simulink model "model_my_paper"  (R2024a)
settings: Solver=FixedStepAuto  StartTime=0.0  StopTime=40  FixedStep=0.01  RelTol=1e-3
undefined symbols (not defined in the file or in its folder): e0_0, e1_0, e2_0, e3_0, q0, vec
libraries: sharedtransform x8, dspsigops x3, aerolibsim3d x2, sharedutil x2, sim3dlib x1, aerolibutil x1
settings Model: Creator=bemran  LastModifiedBy=bemran

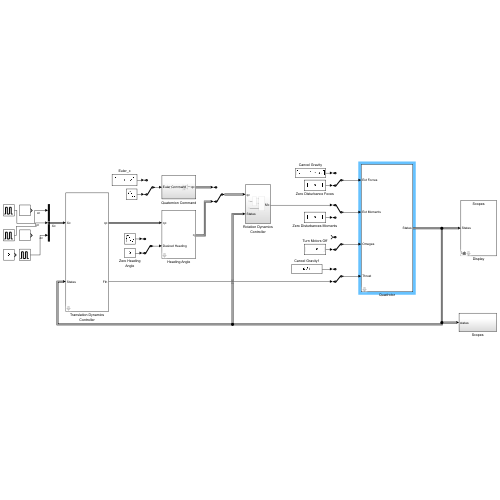
[thumbnail: Simulink's stored preview of the top-level diagram]
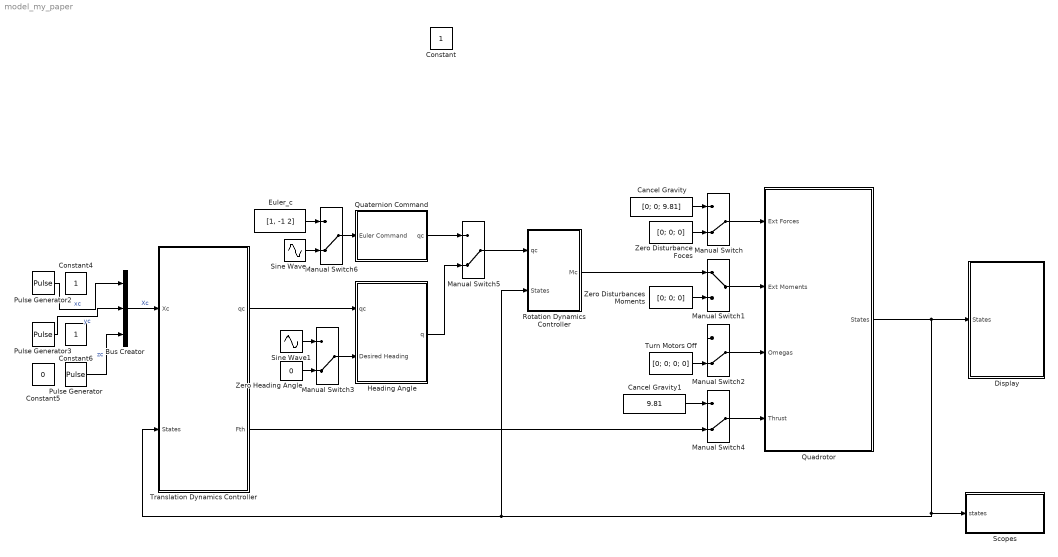
== system model_my_paper ==
  Bus Creator : BusCreator  Inputs=3
  Cancel Gravity : Constant  Value=[0; 0; 9.81]
  Cancel Gravity1 : Constant  Value=9.81
  Constant4 : Constant
  Constant5 : Constant  Value=0
  Constant6 : Constant
  Display : Subsystem  Variant=on  VariantControlMode=label  LabelModeActiveChoice=scopes  mask{VChoice=scopes}
      mask prompts: VChoice "Select method of display"
      mask init:
      | vssBlk = gcb;
      | choice = get_param(vssBlk,'VChoice');
      | if strcmp(choice,'animation')
      |     set_param(vssBlk, 'LabelModeActiveChoice', 'animation');
      | else
      |     set_param(vssBlk, 'LabelModeActiveChoice', 'scopes');
      | end
  Euler_c : Constant  Value=[1, -1 2]
  Heading Angle : Subsystem  mask{FallingSlewLimit=-1, HeadingRisingSlewLimit=1}
      mask prompts: FallingSlewLimit "Heading Falling Slew Limit"; HeadingRisingSlewLimit "Heading Rising Slew Limit"
      mask TypeOptions FallingSlewLimit: Rate Limiter/FallingSlewLimit
      mask TypeOptions HeadingRisingSlewLimit: Rate Limiter/RisingSlewLimit
  Manual Switch{,2..6} (6 alike) : ManualSwitch  CurrentSetting=0
  Manual Switch1 : ManualSwitch
  Pulse Generator : DiscretePulseGenerator  PulseType=Time based  Amplitude=-4  Period=20  PulseWidth=50
  Pulse Generator2 : DiscretePulseGenerator  PulseType=Time based  Amplitude=5  Period=30  PulseWidth=50  PhaseDelay=10
  Pulse Generator3 : DiscretePulseGenerator  PulseType=Time based  Amplitude=-3  Period=30  PulseWidth=50  PhaseDelay=-10
  Quadrotor : Subsystem  mask{mass=1, InertiaMatrix=eye(3), thrust_coff=1, drag_coff=0.1, arm_length=0.3, VelocityBodyInitialValues=zeros(3,1), PositionReferenceInitialValues=zeros(3,1), OmegaInitialValues=zeros(3,1), EulerInitialValues=zeros(3,1)}
      mask prompts: InertiaMatrix "Inertia Matrix"; thrust_coff "Thrust Coefficient"; drag_coff "Drag Coefficient"; arm_length "Arm Length"; VelocityBodyInitialValues "Velocity Body Initial Values"; PositionReferenceInitialValues "Position Reference Initial Values"; OmegaInitialValues "Omega Initial Values"; EulerInitialValues "Euler Initial Values"
      mask TypeOptions mass: 6DOF NWU Mixed/mass
      mask TypeOptions InertiaMatrix: 6DOF NWU Mixed/InertiaMatrix
      mask TypeOptions thrust_coff: Mixer/thrust_coff
      mask TypeOptions drag_coff: Mixer/drag_coff
      mask TypeOptions arm_length: Mixer/arm_length
      mask TypeOptions VelocityBodyInitialValues: 6DOF NWU Mixed/VelocityBodyInitialValues
      mask TypeOptions PositionReferenceInitialValues: 6DOF NWU Mixed/PositionReferenceInitialValues
      mask TypeOptions OmegaInitialValues: 6DOF NWU Mixed/OmegaInitialValues
      mask TypeOptions EulerInitialValues: 6DOF NWU Mixed/EulerInitialValues
  Quaternion Command : Subsystem
  Rotation Dynamics Controller : Subsystem
  Scopes : Subsystem  VariantControl=scopes
  Sine Wave : Sin  Amplitude=[1*pi;1*pi; 1*pi]  Frequency=[0.1, 0.05, 0.02]  Phase=[pi/6, pi/2, -pi/6]  SampleTime=0
  Sine Wave1 : Sin  Amplitude=2*pi  Frequency=0.1  SampleTime=0
  Translation Dynamics Controller : Subsystem
      mask DialogControl ParameterGroupVar Prompt: Desired Signal
      mask DialogControl Container3 Prompt: Control Signal
  Turn Motors Off : Constant  Value=[0; 0; 0; 0]
  Zero Disturbance Foces : Constant  Value=[0; 0; 0]
  Zero Disturbances Moments : Constant  Value=[0; 0; 0]
  Zero Heading Angle : Constant  Value=0
  Constant : Constant  IOType=siggen
  wires:
  Quadrotor/1(States) -> Rotation Dynamics Controller/2(States), Translation Dynamics Controller/2(States), Scopes/1(states), Display/1(States)
  Zero Disturbance Foces/1 -> Manual Switch/2
  Manual Switch/1 -> Quadrotor/1(Ext Forces)
  Zero Disturbances Moments/1 -> Manual Switch1/2
  Manual Switch1/1 -> Quadrotor/2(Ext Moments)
  Manual Switch2/1 -> Quadrotor/3(Omegas)
  Turn Motors Off/1 -> Manual Switch2/2
  Pulse Generator2/1 -> Bus Creator/1  "xc"
  Pulse Generator/1 -> Bus Creator/3  "zc"
  Pulse Generator3/1 -> Bus Creator/2  "yc"
  Cancel Gravity/1 -> Manual Switch/1
  Manual Switch4/1 -> Quadrotor/4(Thrust)
  Cancel Gravity1/1 -> Manual Switch4/1
  Rotation Dynamics Controller/1(Mc) -> Manual Switch1/1
  Manual Switch5/1 -> Rotation Dynamics Controller/1(qc)
  Quaternion Command/1(qc) -> Manual Switch5/1
  Bus Creator/1 -> Translation Dynamics Controller/1(Xc)  "Xc"
  Translation Dynamics Controller/2(Fth) -> Manual Switch4/2
  Manual Switch3/1 -> Heading Angle/2(Desired Heading)
  Heading Angle/1(q) -> Manual Switch5/2
  Sine Wave1/1 -> Manual Switch3/1
  Zero Heading Angle/1 -> Manual Switch3/2
  Manual Switch6/1 -> Quaternion Command/1(Euler Command)
  Sine Wave/1 -> Manual Switch6/2
  Euler_c/1 -> Manual Switch6/1
  Translation Dynamics Controller/1(qc) -> Heading Angle/1(qc)

== system model_my_paper/Display ==
  States : Inport
  Animation : Subsystem  VariantControl=animation
  Scopes : Subsystem  VariantControl=scopes

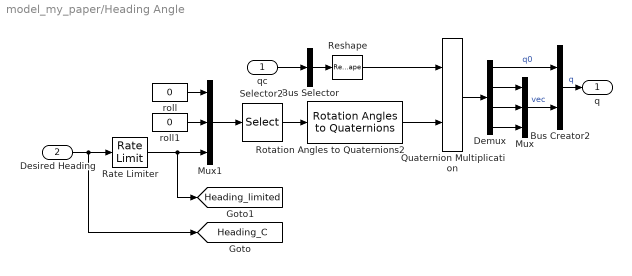
== system model_my_paper/Heading Angle ==
  qc : Inport
  Desired Heading : Inport  Port=2
  Bus Creator2 : BusCreator  Inputs=q0,vec  OutDataTypeStr=Bus: QuaturnionBus
  Bus Selector : BusSelector  OutputSignals=q0,vec  OutputAsBus=on
  Demux : Demux
  Mux : Mux  Inputs=3
  Mux1 : Mux  Inputs=3
  Quaternion Multiplication : aerolibutil/Quaternion Multiplication
  Rate Limiter : RateLimiter  RisingSlewLimit=HeadingRisingSlewLimit  FallingSlewLimit=FallingSlewLimit  SampleTimeMode=inherited
  Reshape : Reshape
  Rotation Angles to Quaternions2 : sharedtransform/Rotation Angles to Quaternions  rotationOrder=ZYX  aMode=aMode
  Selector2 : Selector  InputPortWidth=3  IndexOptions=Index vector (dialog)  Indices=[3 2 1]  OutputSizes=1
  roll : Constant  Value=0
  roll1 : Constant  Value=0
  q : Outport
  tag scope: Heading_C=global, Heading_limited=global
  wires:
  Selector2/1 -> Rotation Angles to Quaternions2/1
  Demux/1 -> Bus Creator2/1  "q0"
  Mux/1 -> Bus Creator2/2  "vec"
  Bus Selector/1 -> Reshape/1
  Quaternion Multiplication/1 -> Demux/1
  Rotation Angles to Quaternions2/1 -> Quaternion Multiplication/2
  Demux/2 -> Mux/1
  Bus Creator2/1 -> q/1  "q"
  Demux/4 -> Mux/3
  Reshape/1 -> Quaternion Multiplication/1
  Demux/3 -> Mux/2
  Mux1/1 -> Selector2/1
  qc/1 -> Bus Selector/1
  Rate Limiter/1 -> [Heading_limited], Mux1/3
  roll/1 -> Mux1/1
  roll1/1 -> Mux1/2
  Desired Heading/1 -> [Heading_C], Rate Limiter/1

== system model_my_paper/Quadrotor ==
  Ext Forces : Inport
  Ext Moments : Inport  Port=2
  Omegas : Inport  Port=3
  Thrust : Inport  Port=4
  6DOF NWU Mixed : Subsystem  mask{InertiaMatrix=InertiaMatrix, mass=mass, VelocityBodyInitialValues=VelocityBodyInitialValues, PositionReferenceInitialValues=PositionReferenceInitialValues, OmegaInitialValues=OmegaInitialValues, EulerInitialValues=EulerInitialValues}
      mask prompts: InertiaMatrix "Inertia Matrix"; VelocityBodyInitialValues "Velocity Body Initial Values"; PositionReferenceInitialValues "Position Reference Initial Values"; OmegaInitialValues "Omega Initial Values"; EulerInitialValues "Euler Initial Values"
      mask TypeOptions InertiaMatrix: Angular Velocity Dyanmics/InertiaMatrix
      mask TypeOptions mass: Translation Dynamics/mass
      mask TypeOptions VelocityBodyInitialValues: Translation Dynamics/VelocityBodyInitialValues
      mask TypeOptions PositionReferenceInitialValues: Translation Dynamics/PositionReferenceInitialValues
      mask TypeOptions OmegaInitialValues: Angular Velocity Dyanmics/OmegaInitialValues
      mask TypeOptions EulerInitialValues: Quaternion Dynamics/EulerInitialValues
      mask DialogControl Parameters Prompt: Parameters
      mask DialogControl Container6 Prompt: Initial Values
  Bus Selector : BusSelector  OutputSignals=DCM_be
  Forces in Inertia frame : Subsystem  mask{mass=mass, Gravity=9.81}
  Mixer : Subsystem  mask{thrust_coff=thrust_coff, drag_coff=drag_coff, arm_length=arm_length}
      mask prompts: thrust_coff "Thrust Coefficient"; drag_coff "Drag Coefficient"; arm_length "Arm Length"
  Moments in Body frame : Subsystem
  States : Outport
  tag scope: Fe=global, Mb=global
  wires:
  6DOF NWU Mixed/1(States) -> States/1, Bus Selector/1
  Forces in Inertia frame/1(Fe) -> [Fe], 6DOF NWU Mixed/1(Fe)
  Bus Selector/1 -> Forces in Inertia frame/2(DCM_be)  "<DCM_be>"
  Omegas/1 -> Mixer/1(Omegas)
  Thrust/1 -> Forces in Inertia frame/3(Thrust)
  Mixer/2(Torques) -> Moments in Body frame/2(Torque)
  Ext Moments/1 -> Moments in Body frame/1(Ext Moments)
  Ext Forces/1 -> Forces in Inertia frame/1(Ext Forces)
  Moments in Body frame/1(Mb) -> [Mb], 6DOF NWU Mixed/2(Moments)

== system model_my_paper/Quaternion Command ==
  Euler Command : Inport
  Bus Creator1 : BusCreator  Inputs=2  OutDataTypeStr=Bus: QuaturnionBus
  Demux1 : Demux
  Mux1 : Mux  Inputs=3
  Rotation Angles to Quaternions : sharedtransform/Rotation Angles to Quaternions  rotationOrder=ZYX  aMode=aMode
  Selector : Selector  InputPortWidth=3  IndexOptions=Index vector (dialog)  Indices=[3 2 1]  OutputSizes=1
  qc : Outport  OutDataTypeStr=Bus: QuaturnionBus  PortDimensions=1
  wires:
  Selector/1 -> Rotation Angles to Quaternions/1
  Euler Command/1 -> Selector/1
  Demux1/3 -> Mux1/2
  Rotation Angles to Quaternions/1 -> Demux1/1
  Demux1/2 -> Mux1/1
  Demux1/4 -> Mux1/3
  Demux1/1 -> Bus Creator1/1  "q0"
  Mux1/1 -> Bus Creator1/2  "vec"
  Bus Creator1/1 -> qc/1  "q"

== system model_my_paper/Rotation Dynamics Controller ==
  qc : Inport  OutDataTypeStr=Bus: QuaturnionBus
  States : Inport  Port=2
  My paper controller : Subsystem  mask{RotationControlGain=eye(3) * 9, AngularRateControlGain=eye(3) * 10, DesiredAngularRateInitialCondition=[0;0;0]}
      mask prompts: RotationControlGain "Rotation Control Gain"; AngularRateControlGain "Angular Rate Control Gain"; DesiredAngularRateInitialCondition "Desired Angular Rate Initial Condition"
      mask TypeOptions RotationControlGain: Kr/Value
      mask TypeOptions AngularRateControlGain: Kw/Value
      mask TypeOptions DesiredAngularRateInitialCondition:
      | Desired Angular
      | Rate Integaration/InitialCondition
      mask DialogControl ParameterGroupVar Prompt: Control Gain
      mask DialogControl Container3 Prompt: Initail Condition
  Quaternion Dynamics : Subsystem  mask{QuaternionAngleDynamicGain=30, QuaternionInitialCondition=[1;0;0;0], DesiredRotaionDynamciGain=30}
      mask prompts: QuaternionAngleDynamicGain "Quaternion Angle Dynamic Gain"; QuaternionInitialCondition "Quaternion Initial Condition"; DesiredRotaionDynamciGain "Desired Rotaion Dynamci Gain"
      mask TypeOptions QuaternionAngleDynamicGain:
      | Quaternion Angle
      | Dynamic Gain/Gain
      mask TypeOptions QuaternionInitialCondition:
      | Quaternion
      | Integration/InitialCondition
      mask TypeOptions DesiredRotaionDynamciGain:
      | Desired Rotaion
      | Dynamic Gain /Gain
  Mc : Outport
  wires:
  qc/1 -> Quaternion Dynamics/1(qc)
  Quaternion Dynamics/1(Rd) -> My paper controller/1(Rd)
  My paper controller/1(Mc) -> Mc/1
  States/1 -> My paper controller/3(States)
  Quaternion Dynamics/2(Rd_dot) -> My paper controller/2(Rd_dot)

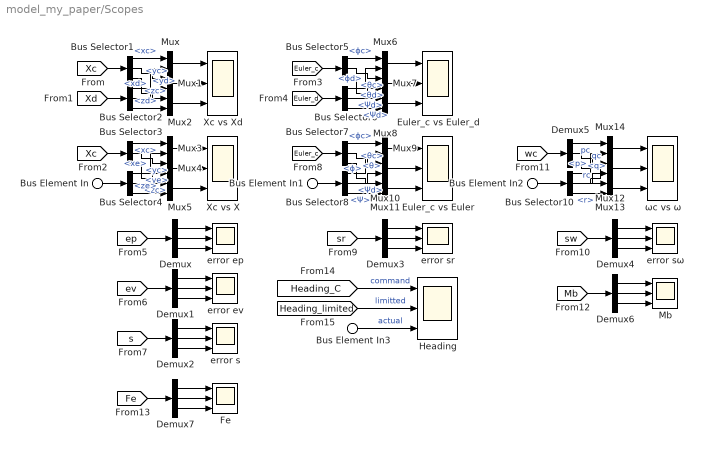
== system model_my_paper/Scopes ==
  Bus Element In : Inport  PortName=states  Element=Xe
  Bus Element In1 : Inport  PortName=states  Element=Euler
  Bus Element In3 : Inport  PortName=states  Element=Euler.Ψ
  Bus Element In2 : Inport  PortName=states  Element=ω
  Bus Selector1 : BusSelector  OutputSignals=xc,yc,zc
  Bus Selector10 : BusSelector  OutputSignals=p,q,r
  Bus Selector2 : BusSelector  OutputSignals=pose.xd,pose.yd,pose.zd
  Bus Selector3 : BusSelector  OutputSignals=xc,yc,zc
  Bus Selector4 : BusSelector  OutputSignals=xe,ye,ze
  Bus Selector5 : BusSelector  OutputSignals=ϕc,θc,Ψd
  Bus Selector6 : BusSelector  OutputSignals=ϕd,θd,Ψd
  Bus Selector7 : BusSelector  OutputSignals=ϕc,θc,Ψd
  Bus Selector8 : BusSelector  OutputSignals=ϕ,θ,Ψ
  Demux{,1..7} (8 alike) : Demux  Outputs=3
  Euler_c vs Euler : Scope  NumInputPorts=3
  Euler_c vs Euler_d : Scope  NumInputPorts=3
  Fe : Scope  NumInputPorts=3
  Heading : Scope  NumInputPorts=3
  Mb : Scope  NumInputPorts=3
  Mux{,1..14} (15 alike) : Mux  Inputs=2
  Xc vs X : Scope  NumInputPorts=3
  Xc vs Xd : Scope  NumInputPorts=3
  error ep : Scope  NumInputPorts=3
  error ev : Scope  NumInputPorts=3
  error s : Scope  NumInputPorts=3
  error sr : Scope  NumInputPorts=3
  error sω : Scope  NumInputPorts=3
  ωc vs ω : Scope  NumInputPorts=3
  wires:
  [Xc] -> Bus Selector1/1
  [Xd] -> Bus Selector2/1
  Bus Selector1/1 -> Mux/1  "<xc>"
  Bus Selector2/1 -> Mux/2  "<xd>"
  Bus Selector2/3 -> Mux2/2  "<zd>"
  Bus Selector2/2 -> Mux1/2  "<yd>"
  Bus Selector1/3 -> Mux2/1  "<zc>"
  Bus Selector1/2 -> Mux1/1  "<yc>"
  Mux/1 -> Xc vs Xd/1
  Mux1/1 -> Xc vs Xd/2
  Mux2/1 -> Xc vs Xd/3
  Mux5/1 -> Xc vs X/3
  Mux4/1 -> Xc vs X/2
  Mux3/1 -> Xc vs X/1
  Bus Selector3/2 -> Mux4/1  "<yc>"
  Bus Selector3/3 -> Mux5/1  "<zc>"
  Bus Selector4/2 -> Mux4/2  "<ye>"
  Bus Selector4/3 -> Mux5/2  "<ze>"
  Bus Selector4/1 -> Mux3/2  "<xe>"
  Bus Selector3/1 -> Mux3/1  "<xc>"
  Bus Element In/1 -> Bus Selector4/1
  [Xc] -> Bus Selector3/1
  Mux8/1 -> Euler_c vs Euler_d/3
  Mux7/1 -> Euler_c vs Euler_d/2
  Mux6/1 -> Euler_c vs Euler_d/1
  Bus Selector5/2 -> Mux7/1  "<θc>"
  Bus Selector5/3 -> Mux8/1  "<Ψd>"
  Bus Selector6/2 -> Mux7/2  "<θd>"
  Bus Selector6/3 -> Mux8/2  "<Ψd>"
  Bus Selector6/1 -> Mux6/2  "<ϕd>"
  Bus Selector5/1 -> Mux6/1  "<ϕc>"
  [Euler_d] -> Bus Selector6/1
  [Euler_c] -> Bus Selector5/1
  [ep] -> Demux/1
  Demux/1 -> error ep/1
  Demux/2 -> error ep/2
  Demux/3 -> error ep/3
  Demux1/3 -> error ev/3
  Demux1/2 -> error ev/2
  [ev] -> Demux1/1
  Demux1/1 -> error ev/1
  [s] -> Demux2/1
  Demux2/2 -> error s/2
  Demux2/3 -> error s/3
  Demux2/1 -> error s/1
  [Euler_c] -> Bus Selector7/1
  Bus Element In1/1 -> Bus Selector8/1
  Bus Selector7/1 -> Mux9/1  "<ϕc>"
  Bus Selector8/1 -> Mux9/2  "<ϕ>"
  Bus Selector8/3 -> Mux11/2  "<Ψ>"
  Bus Selector8/2 -> Mux10/2  "<θ>"
  Bus Selector7/3 -> Mux11/1  "<Ψd>"
  Bus Selector7/2 -> Mux10/1  "<θc>"
  Mux9/1 -> Euler_c vs Euler/1
  Mux10/1 -> Euler_c vs Euler/2
  Mux11/1 -> Euler_c vs Euler/3
  Demux4/1 -> error sω/1
  [sw] -> Demux4/1
  Demux4/2 -> error sω/2
  Demux4/3 -> error sω/3
  Demux3/3 -> error sr/3
  Demux3/2 -> error sr/2
  Demux3/1 -> error sr/1
  [sr] -> Demux3/1
  Mux13/1 -> ωc vs ω/3
  Mux12/1 -> ωc vs ω/2
  Mux14/1 -> ωc vs ω/1
  Demux5/2 -> Mux12/1  "qc"
  Demux5/3 -> Mux13/1  "rc"
  Bus Selector10/2 -> Mux12/2  "<q>"
  Bus Selector10/3 -> Mux13/2  "<r>"
  Bus Selector10/1 -> Mux14/2  "<p>"
  Demux5/1 -> Mux14/1  "pc"
  Bus Element In2/1 -> Bus Selector10/1
  [wc] -> Demux5/1
  Demux6/3 -> Mb/3
  Demux6/2 -> Mb/2
  [Mb] -> Demux6/1
  Demux6/1 -> Mb/1
  Demux7/1 -> Fe/1
  [Fe] -> Demux7/1
  Demux7/2 -> Fe/2
  Demux7/3 -> Fe/3
  Bus Element In3/1 -> Heading/3  "actual"
  [Heading_limited] -> Heading/2  "limitted"
  [Heading_C] -> Heading/1  "command"

== system model_my_paper/Translation Dynamics Controller ==
  Xc : Inport
  States : Inport  Port=2
  Desired Position Dynamcis : Subsystem  mask{RisingSlewLimit=[1;1;1] * 3, FallingSlewLimit=[-1;-1;-1] * 3, DesiredVelocityDynamicGain=[1;1;1] * 6, DesiredPositionDynamicGain=[1;1;1] * 8, DesiredPositionInitialCondition=zeros(3,1), DesiredVelocityInitialCondition=zeros(3,1)}
      mask prompts: RisingSlewLimit "Simulink:blkprm_prompts:RateLimRisingSlewRate"; FallingSlewLimit "Simulink:blkprm_prompts:RateLimFallingSlewRate"; DesiredVelocityDynamicGain "Desired Velocity Dynamic Gain"; DesiredPositionDynamicGain "Desired Position Dynamic Gain"; DesiredPositionInitialCondition "Desired Position Initial Condition"; DesiredVelocityInitialCondition "Desired Velocity Initial Condition"
      mask TypeOptions RisingSlewLimit: Rate Limiter/RisingSlewLimit
      mask TypeOptions FallingSlewLimit: Rate Limiter/FallingSlewLimit
      mask TypeOptions DesiredVelocityDynamicGain:
      | Desired Velocity
      | Dynamic Gain/Gain
      mask TypeOptions DesiredPositionDynamicGain:
      | Desired Position
      | Dynamic Gain/Gain
      mask TypeOptions DesiredPositionInitialCondition:
      | Position
      | Integration/InitialCondition
      mask TypeOptions DesiredVelocityInitialCondition:
      | Velocity
      | Integration/InitialCondition
      mask DialogControl ParameterGroupVar Prompt: Slew rate for change in position
      mask DialogControl RisingSlewLimit Prompt: Rising slew rate:
      mask DialogControl FallingSlewLimit Prompt: Falling slew rate:
      mask DialogControl Container4 Prompt: Initial values
  My paper Translation Controller but for Quaternion : Subsystem  mask{PositionErrorGain=eye(3) * 3, VelocityErrorGain=eye(3) * 4}
      mask prompts: PositionErrorGain "Position Error Gain"; VelocityErrorGain "Velocity Error Gain"
      mask TypeOptions PositionErrorGain: Kx/Value
      mask TypeOptions VelocityErrorGain: Kv/Value
      mask DialogControl ParameterGroupVar Prompt: Control Parameters
  qc : Outport  OutDataTypeStr=Bus: QuaturnionBus
  Fth : Outport  Port=2
  tag scope: Xc=global, Xd=global
  wires:
  Desired Position Dynamcis/1(Xd) -> [Xd], My paper Translation Controller but for Quaternion/1(Xd)
  States/1 -> My paper Translation Controller but for Quaternion/2(States)
  My paper Translation Controller but for Quaternion/2(Fth) -> Fth/1
  Xc/1 -> [Xc], Desired Position Dynamcis/1(Desired Position)
  My paper Translation Controller but for Quaternion/1(qc) -> qc/1

== system model_my_paper/Display/Animation ==
  States : Inport
  Bus Selector : BusSelector  OutputSignals=Xe,Euler
  Simulation 3D Multirotor Pack : aerolibsim3d/Simulation 3D Multirotor Pack  Rotor1_T=off  Rotor1_R=off  Rotor2_T=off  Rotor2_R=off  Rotor3_T=off  Rotor3_R=off  Rotor4_T=off  Rotor4_R=off  Rotor5_T=off  Rotor5_R=off  Rotor6_T=off  Rotor6_R=off  Rotor7_T=off  Rotor7_R=off  Rotor8_T=off  Rotor8_R=off  Sensor1_T=off  Sensor1_R=off  Sensor2_T=off  Sensor2_R=off  GeoRadioButton=NED  AdjustForCesium=off  Heading0=90
  Simulation 3D Rotorcraft : aerolibsim3d/Simulation 3D Rotorcraft  Priority=-1  Mesh=Multirotor  MeshPath=/MathWorksAerospaceContent/Vehicles/Rotorcraft/Helicopter/Mesh/SK_Helicopter.SK_Helicopter  MeshPathLight=/MathWorksAerospaceContent/Vehicles/Rotorcraft/LightHelicopter/Mesh/SK_LightHelicopter.SK_LightHelicopter  MeshPathMulti=/MathWorksAerospaceContent/Vehicles/Rotorcraft/Multirotor/Mesh/SK_Quadcopter.SK_Quadcopter  AircraftColor=Red  ActorName=SimulinkVehicle3  Translation=zeros(11, 3)  Rotation=zeros(11, 3)  IsGHSensorEnabled=off  AreGHRaysVisible=on  IsOutputReshapeEnabled=off  GHRayLength=1524  GHBodyOffset=1.169  GHFrontTireRadius=0.196  GHLeftTireRadius=0.203  GHRightTireRadius=0.203  GHContactLocation1=[1.47 -1.04 1.169]  GHContactLocation2=[-1.24 -1.04 1.169]  GHContactLocation3=[-1.24 1.04 1.169]  GHContactLocation4=[1.47 1.04 1.169]  WoWSensorTolerance=0.05  LightsConfig=Automatic lights  LandingLightIntensity=300000  LandingLightConeAngle=15  LandingLightColor=[1 1 1]  HelicopterLeftLandingLightLocation=[0 0 0]  HelicopterLeftLandingLightOrientation=[0 0 0]  NoseLightIntensity=150000  NoseLightConeAngle=36  HelicopterNoseLightLocation=[0 0 0]  HelicopterNoseLightOrientation=[0 0 0]  NavLightIntensity=500  PositionLightIntensity=500  StrobeLightIntensity=5000  StrobeLightColor=[1 1 1]  StrobePeriod=1.5  StrobePulseWidth=6  BeaconLightIntensity=4000  BeaconLightColor=[1 0 0]  BeaconPeriod=1.5  BeaconPulseWidth=10  SampleTime=0.1  ActorType=SimulinkVehicle  ID=3  aMode=0  ActorTag=SimulinkVehicle3
  Simulation 3D Scene Configuration1 : sim3dlib/Simulation 3D Scene Configuration  Priority=0  ProjectFormat=Default Scenes  SceneDesc=Airport  ProjectName=C:\Program Files\MATLAB\R2024a\toolbox\shared\sim3d_projects\automotive_project_windows\UE\WindowsNoEditor\VehicleSimulation.exe  ScenePath=/Game/Maps/HwStrght  EnableOpenDRIVE=off  vehTagList={'Scene Origin';'SimulinkVehicle2';'SimulinkVehicle3'}  vehTag=SimulinkVehicle2  FreeCameraInitialTranslation=[-6, 0, 2]  FreeCameraDefaultInitialTranslation=[-6, 0, 2]  FreeCameraInitialRotation=[0, -15, 0]  FreeCameraDefaultInitialRotation=[0, -15, 0]  OpVisEn=off  Ts=.1  EnableWindow=on  EnableRemoteAccess=off  EnableWeather=off  SunAzimuth=90  SunAltitude=40.0  EnableGeospatialSun=off  Latitude=0  Longitude=0  Date=2023-01-01  Time=10:30:00  GeoTimeZone=-5.0  SunDaylightSaving=off  wind=1  clouds=10  EnableVolumetricClouds=off  CloudCoverage=0  CloudAltitude=6  fog=0  rain=0  RaindropsEffect=off  SnowDensity=0  EnableGeospatial=off  UseTrueOrigin=off  OriginHeight=200  OriginLatitude=40.744652  OriginLongitude=-73.988864  MapStyle=Aerial  AdditionalAssetIDs=[]  UseAdvancedSunSky=off  SolarTime=11  TimeZone=-5  Day=21  Month=9  Year=2022  UseDaylightSavingTime=on  DSTStartDay=10  DSTStartMonth=3  DSTEndDay=3  DSTEndMonth=11  DSTSwitchHour=2  sensorTag=MainCamera1  sensorId=1  sensorName=MainCamera1  mountLoc=Origin  offsetFlag=off  tmountOffset=[0, 0, 0]  rmountOffset=[0, 0, 0]  HorizontalResolution=1280  VerticalResolution=720  HorizontalFOV=60  mountPoint=[0 0 0]  mountOrientation=[0 0 0]  aMode=0  ID=1  GeoTrigger=Inactive
      settings: LibrarySourceBlock=aerolibsim3d/Simulation 3D Scene Configuration
  wires:
  Simulation 3D Multirotor Pack/1 -> Simulation 3D Rotorcraft/1
  Simulation 3D Multirotor Pack/2 -> Simulation 3D Rotorcraft/2
  Bus Selector/1 -> Simulation 3D Multirotor Pack/1  "<Xe>"
  Bus Selector/2 -> Simulation 3D Multirotor Pack/2  "<Euler>"
  States/1 -> Bus Selector/1

== system model_my_paper/Display/Scopes ==
  States : Inport
  Bus Selector : BusSelector  OutputSignals=Xe,Euler
  Demux : Demux  Outputs=3
  Demux1 : Demux  Outputs=3
  Scope : Scope  NumInputPorts=3
  Scope1 : Scope  NumInputPorts=3
  wires:
  Demux/1 -> Scope/1
  Demux/2 -> Scope/2
  Demux/3 -> Scope/3
  Demux1/1 -> Scope1/1
  Demux1/2 -> Scope1/2
  Demux1/3 -> Scope1/3
  Bus Selector/2 -> Demux1/1  "<Euler>"
  Bus Selector/1 -> Demux/1  "<Xe>"
  States/1 -> Bus Selector/1

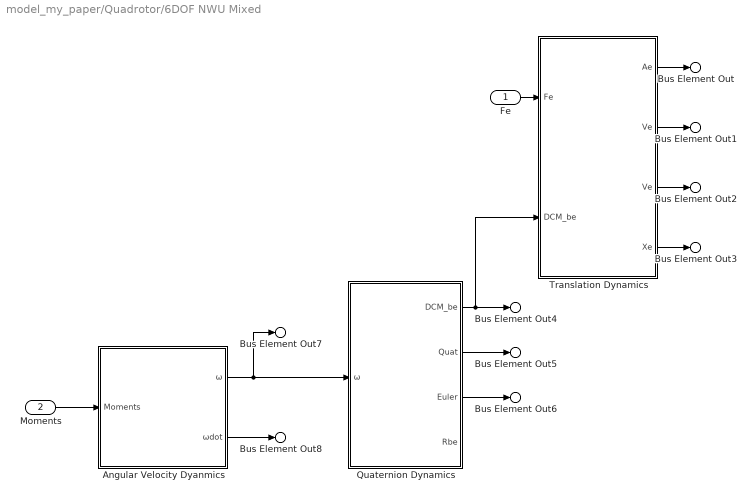
== system model_my_paper/Quadrotor/6DOF NWU Mixed ==
  Fe : Inport  OutDataTypeStr=double  Unit=N  PortDimensions=3
  Moments : Inport  Port=2  OutDataTypeStr=double
  Angular Velocity Dyanmics : Subsystem  mask{OmegaInitialValues=OmegaInitialValues, InertiaMatrix=InertiaMatrix}
      mask prompts: OmegaInitialValues "Omega Initial Values"; InertiaMatrix "Inertia Matrix"
  Quaternion Dynamics : Subsystem  mask{EulerInitialValues=EulerInitialValues}
      mask prompts: EulerInitialValues "Euler Initial Values"
  Translation Dynamics : Subsystem  mask{mass=mass, gravity=9.81, VelocityBodyInitialValues=VelocityBodyInitialValues, PositionReferenceInitialValues=PositionReferenceInitialValues}
      mask prompts: gravity "Gravity (m/s2)"; VelocityBodyInitialValues "Velocity Body Initial Values"; PositionReferenceInitialValues "Position Reference Initial Values"
  Bus Element Out : Outport  PortName=States  Element=Ae
  Bus Element Out1 : Outport  PortName=States  Element=Vb
  Bus Element Out2 : Outport  PortName=States  Element=Ve
  Bus Element Out3 : Outport  PortName=States  Element=Xe
  Bus Element Out4 : Outport  PortName=States  Element=DCM_be
  Bus Element Out5 : Outport  PortName=States  Element=Quat
  Bus Element Out6 : Outport  PortName=States  Element=Euler
  Bus Element Out7 : Outport  PortName=States  Element=ω
  Bus Element Out8 : Outport  PortName=States  Element=ωdot
  wires:
  Quaternion Dynamics/1(DCM_be) -> Translation Dynamics/2(DCM_be), Bus Element Out4/1
  Angular Velocity Dyanmics/2(ωdot) -> Bus Element Out8/1
  Quaternion Dynamics/2(Quat) -> Bus Element Out5/1
  Angular Velocity Dyanmics/1(ω) -> Bus Element Out7/1, Quaternion Dynamics/1(ω)
  Translation Dynamics/3(Ve) -> Bus Element Out2/1
  Moments/1 -> Angular Velocity Dyanmics/1(Moments)
  Quaternion Dynamics/3(Euler) -> Bus Element Out6/1
  Translation Dynamics/2("Ve ") -> Bus Element Out1/1
  Translation Dynamics/4(Xe) -> Bus Element Out3/1
  Translation Dynamics/1(Ae) -> Bus Element Out/1
  Fe/1 -> Translation Dynamics/1(Fe)

== system model_my_paper/Quadrotor/Forces in Inertia frame ==
  Ext Forces : Inport
  DCM_be : Inport  Port=2
  Thrust : Inport  Port=3
  Gravity Force in Inertia Frame : Subsystem
  Reshape1 : Reshape  OutputDimensionality=Column vector (2-D)
  Reshape2 : Reshape
  Sum : Sum  Inputs=+++
  Thrust in Inertia Frame : Subsystem
  Fe : Outport
  wires:
  Gravity Force in Inertia Frame/1(Ge) -> Sum/2
  Reshape1/1 -> Sum/1
  Reshape2/1 -> Fe/1
  Ext Forces/1 -> Reshape1/1
  Sum/1 -> Reshape2/1
  DCM_be/1 -> Thrust in Inertia Frame/1(DCM_be)
  Thrust in Inertia Frame/1(Te) -> Sum/3
  Thrust/1 -> Thrust in Inertia Frame/2(Thrust)

== system model_my_paper/Quadrotor/Mixer ==
  Omegas : Inport
  Bus Creator : BusCreator  Inputs=3
  Fcn : Fcn  Expr=u(1) + u(2) + u(3) + u(4)
  Fcn1 : Fcn  Expr=-u(1) + u(3)
  Fcn2 : Fcn  Expr=-u(2) + u(4)
  Fcn3 : Fcn  Expr=u(1) - u(2) + u(3) - u(4)
  Square : Math  Operator=square
  b : Gain  Gain=thrust_coff
  c : Gain  Gain=drag_coff
  l : Gain  Gain=arm_length
  Thrust : Outport
  Torques : Outport  Port=2
  wires:
  b/1 -> Fcn/1, l/1
  l/1 -> Fcn2/1, Fcn1/1
  Omegas/1 -> Square/1
  c/1 -> Fcn3/1
  Fcn/1 -> Thrust/1
  Square/1 -> c/1, b/1
  Bus Creator/1 -> Torques/1
  Fcn1/1 -> Bus Creator/1  "Tx"
  Fcn2/1 -> Bus Creator/2  "Ty"
  Fcn3/1 -> Bus Creator/3  "Tz"

== system model_my_paper/Quadrotor/Moments in Body frame ==
  Ext Moments : Inport
  Torque : Inport  Port=2
  Reshape2 : Reshape
  Sum : Sum  Inputs=+|+
  Mb : Outport
  wires:
  Ext Moments/1 -> Sum/1
  Reshape2/1 -> Mb/1
  Torque/1 -> Sum/2
  Sum/1 -> Reshape2/1

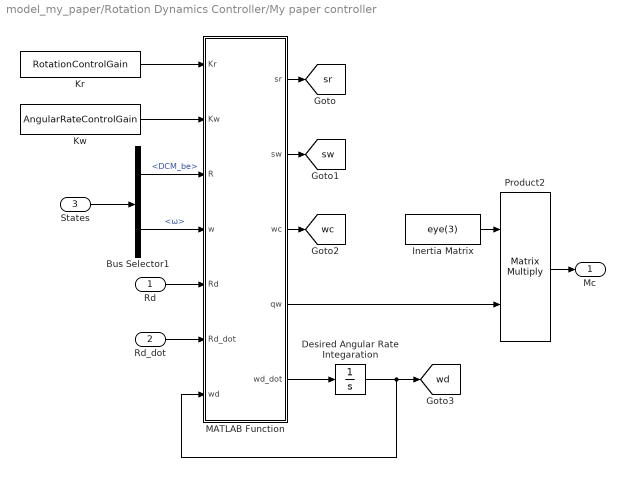
== system model_my_paper/Rotation Dynamics Controller/My paper controller ==
  Rd : Inport
  Rd_dot : Inport  Port=2
  States : Inport  Port=3
  Bus Selector1 : BusSelector  OutputSignals=DCM_be,ω
  Desired Angular Rate Integaration : Integrator  InitialCondition=DesiredAngularRateInitialCondition
  Inertia Matrix : Constant  Value=eye(3)
  Kr : Constant  Value=RotationControlGain
  Kw : Constant  Value=AngularRateControlGain
  MATLAB Function : MATLAB Function  TreatAsAtomicUnit=on
  Product2 : Product  Inputs=**  Multiplication=Matrix(*)  SaturateOnIntegerOverflow=on  OutDataTypeStr=Inherit: Same as first input
  Mc : Outport
  tag scope: sr=global, sw=global, wc=global, wd=global
  wires:
  Bus Selector1/1 -> MATLAB Function/3(R)  "<DCM_be>"
  Kw/1 -> MATLAB Function/2(Kw)
  Bus Selector1/2 -> MATLAB Function/4(w)  "<ω>"
  Rd/1 -> MATLAB Function/5(Rd)
  MATLAB Function/1(sr) -> [sr]
  Kr/1 -> MATLAB Function/1(Kr)
  MATLAB Function/5(wd_dot) -> Desired Angular Rate Integaration/1
  MATLAB Function/3(wc) -> [wc]
  States/1 -> Bus Selector1/1
  Desired Angular Rate Integaration/1 -> [wd], MATLAB Function/7(wd)
  MATLAB Function/4(qw) -> Product2/2
  Inertia Matrix/1 -> Product2/1
  Product2/1 -> Mc/1
  Rd_dot/1 -> MATLAB Function/6(Rd_dot)
  MATLAB Function/2(sw) -> [sw]

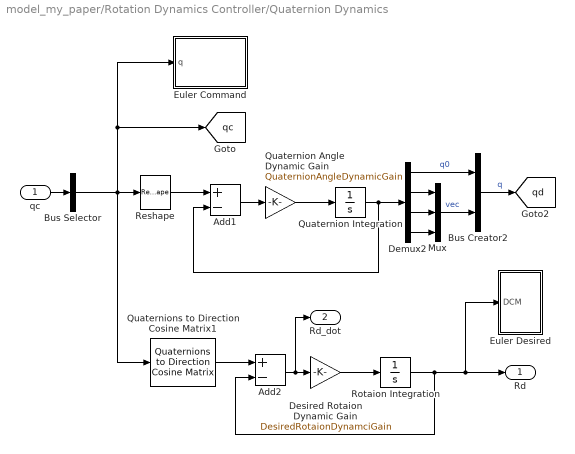
== system model_my_paper/Rotation Dynamics Controller/Quaternion Dynamics ==
  qc : Inport  OutDataTypeStr=Bus: QuaturnionBus
  Add1 : Sum  Inputs=+-
  Add2 : Sum  Inputs=+-
  Bus Creator2 : BusCreator  Inputs=q0,vec  OutDataTypeStr=Bus: QuaturnionBus
  Bus Selector : BusSelector  OutputSignals=q0,vec  OutputAsBus=on
  Demux2 : Demux
  "Desired Rotaion Dynamic Gain " : Gain  Gain=DesiredRotaionDynamciGain
  Euler Command : Subsystem
  Euler Desired : Subsystem
  Mux : Mux  Inputs=3
  Quaternion Integration : Integrator  InitialCondition=QuaternionInitialCondition  ContinuousStateAttributes='qd'
  Quaternion Angle Dynamic Gain : Gain  Gain=QuaternionAngleDynamicGain
  Quaternions to Direction Cosine Matrix1 : sharedtransform/Quaternions to  Direction Cosine Matrix  aMode=aMode
      settings: LibrarySourceBlock=|
      | aerolibtransform2/Quaternions to
      | Direction Cosine Matrix
  Reshape : Reshape  OutputDimensionality=Column vector (2-D)
  Rotaion Integration : Integrator  InitialCondition=eye(3,3)  ContinuousStateAttributes='qd'
  Rd : Outport
  Rd_dot : Outport  Port=2
  tag scope: qc=global, qd=global
  wires:
  Demux2/3 -> Mux/2
  Demux2/2 -> Mux/1
  Quaternion Angle Dynamic Gain/1 -> Quaternion Integration/1
  Demux2/4 -> Mux/3
  Demux2/1 -> Bus Creator2/1  "q0"
  Mux/1 -> Bus Creator2/2  "vec"
  Rotaion Integration/1 -> Add2/2, Euler Desired/1(DCM), Rd/1
  Bus Creator2/1 -> [qd]  "q"
  Quaternion Integration/1 -> Demux2/1, Add1/2
  Add1/1 -> Quaternion Angle Dynamic Gain/1
  qc/1 -> Bus Selector/1
  Reshape/1 -> Add1/1
  Quaternions to Direction Cosine Matrix1/1 -> Add2/1
  Add2/1 -> Rd_dot/1, "Desired Rotaion Dynamic Gain "/1
  "Desired Rotaion Dynamic Gain "/1 -> Rotaion Integration/1
  Bus Selector/1 -> Euler Command/1(q), [qc], Quaternions to Direction Cosine Matrix1/1, Reshape/1

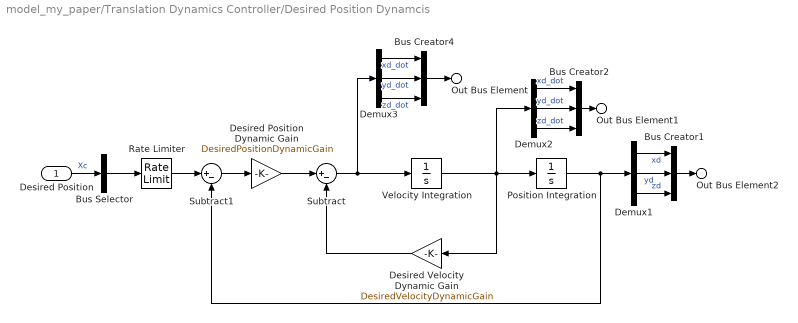
== system model_my_paper/Translation Dynamics Controller/Desired Position Dynamcis ==
  Desired Position : Inport
  Bus Creator1 : BusCreator  Inputs=3
  Bus Creator2 : BusCreator  Inputs=3
  Bus Creator4 : BusCreator  Inputs=3
  Bus Selector : BusSelector  OutputSignals=xc,yc,zc  OutputAsBus=on
  Demux1 : Demux  Outputs=3
  Demux2 : Demux  Outputs=3
  Demux3 : Demux  Outputs=3
  Desired Position Dynamic Gain : Gain  Gain=DesiredPositionDynamicGain
  Desired Velocity Dynamic Gain : Gain  Gain=DesiredVelocityDynamicGain
  Position Integration : Integrator  InitialCondition=DesiredPositionInitialCondition  ContinuousStateAttributes='Xd'
  Rate Limiter : RateLimiter  RisingSlewLimit=RisingSlewLimit  FallingSlewLimit=FallingSlewLimit  SampleTimeMode=inherited
  Subtract : Sum  Inputs=|+-
  Subtract1 : Sum  Inputs=|+-
  Velocity Integration : Integrator  InitialCondition=DesiredVelocityInitialCondition  ContinuousStateAttributes='Vd'
  Out Bus Element2 : Outport  PortName=Xd  Element=pose
  Out Bus Element1 : Outport  PortName=Xd  Element=vel
  Out Bus Element : Outport  PortName=Xd  Element=acc
  wires:
  Bus Creator1/1 -> Out Bus Element2/1
  Bus Selector/1 -> Rate Limiter/1
  Bus Creator2/1 -> Out Bus Element1/1
  Demux1/3 -> Bus Creator1/3  "zd"
  Demux2/2 -> Bus Creator2/2  "yd_dot"
  Demux2/3 -> Bus Creator2/3  "zd_dot"
  Demux2/1 -> Bus Creator2/1  "xd_dot"
  Demux1/1 -> Bus Creator1/1  "xd"
  Demux1/2 -> Bus Creator1/2  "yd"
  Desired Position/1 -> Bus Selector/1  "Xc"
  Subtract/1 -> Demux3/1, Velocity Integration/1
  Velocity Integration/1 -> Demux2/1, Position Integration/1, Desired Velocity Dynamic Gain/1
  Position Integration/1 -> Subtract1/2, Demux1/1
  Desired Velocity Dynamic Gain/1 -> Subtract/2
  Subtract1/1 -> Desired Position Dynamic Gain/1
  Demux3/1 -> Bus Creator4/1  "xd_dot"
  Demux3/2 -> Bus Creator4/2  "yd_dot"
  Demux3/3 -> Bus Creator4/3  "zd_dot"
  Bus Creator4/1 -> Out Bus Element/1
  Rate Limiter/1 -> Subtract1/1
  Desired Position Dynamic Gain/1 -> Subtract/1

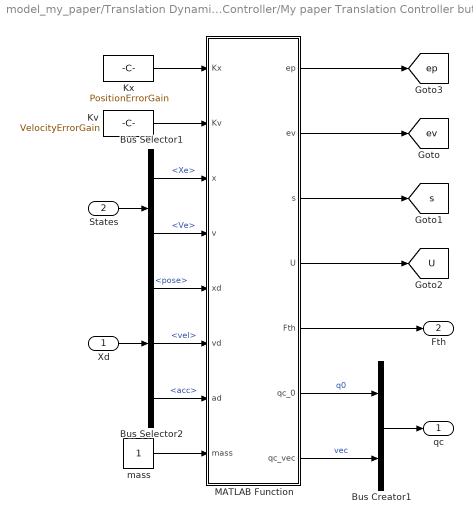
== system model_my_paper/Translation Dynamics Controller/My paper Translation Controller but for Quaternion ==
  Xd : Inport
  States : Inport  Port=2
  Bus Creator1 : BusCreator  Inputs=q0,vec  OutDataTypeStr=Bus: QuaturnionBus
  Bus Selector1 : BusSelector  OutputSignals=Xe,Ve
  Bus Selector2 : BusSelector  OutputSignals=pose,vel,acc
  Kv : Constant  Value=VelocityErrorGain
  Kx : Constant  Value=PositionErrorGain
  MATLAB Function : MATLAB Function  TreatAsAtomicUnit=on
  mass : Constant
  qc : Outport  OutDataTypeStr=Bus: QuaturnionBus  PortDimensions=1
  Fth : Outport  Port=2
  tag scope: U=global, ep=global, ev=global, s=global
  wires:
  States/1 -> Bus Selector1/1
  Kx/1 -> MATLAB Function/1(Kx)
  Bus Selector1/2 -> MATLAB Function/4(v)  "<Ve>"
  Kv/1 -> MATLAB Function/2(Kv)
  Bus Selector1/1 -> MATLAB Function/3(x)  "<Xe>"
  mass/1 -> MATLAB Function/8(mass)
  Xd/1 -> Bus Selector2/1
  Bus Selector2/2 -> MATLAB Function/6(vd)  "<vel>"
  Bus Selector2/1 -> MATLAB Function/5(xd)  "<pose>"
  Bus Selector2/3 -> MATLAB Function/7(ad)  "<acc>"
  MATLAB Function/5(Fth) -> Fth/1
  MATLAB Function/1(ep) -> [ep]
  MATLAB Function/2(ev) -> [ev]
  MATLAB Function/3(s) -> [s]
  MATLAB Function/4(U) -> [U]
  MATLAB Function/7(qc_vec) -> Bus Creator1/2  "vec"
  MATLAB Function/6(qc_0) -> Bus Creator1/1  "q0"
  Bus Creator1/1 -> qc/1

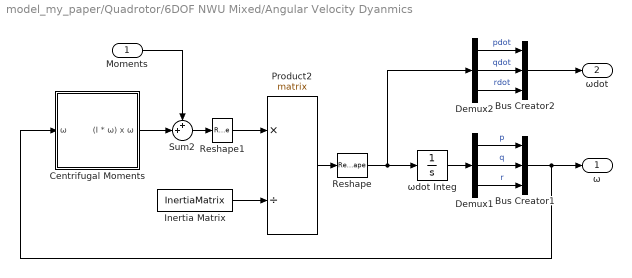
== system model_my_paper/Quadrotor/6DOF NWU Mixed/Angular Velocity Dyanmics ==
  Moments : Inport  OutDataTypeStr=double
  Bus Creator1 : BusCreator  Inputs=3
  Bus Creator2 : BusCreator  Inputs=3
  Centrifugal Moments : Subsystem
  Demux1 : Demux  Outputs=3
  Demux2 : Demux  Outputs=3
  Inertia Matrix : Constant  Value=InertiaMatrix
  Product2 : Product  Inputs=*/  Multiplication=Matrix(*)  SaturateOnIntegerOverflow=on  OutDataTypeStr=Inherit: Same as first input
  Reshape : Reshape
  Reshape1 : Reshape  OutputDimensionality=Row vector (2-D)
  Sum2 : Sum  Inputs=++|  SaturateOnIntegerOverflow=on
  ωdot Integ : Integrator  InitialCondition=OmegaInitialValues  ContinuousStateAttributes={'p', 'q', 'r'}
  ω : Outport
  ωdot : Outport  Port=2  OutDataTypeStr=double  Unit=rad/s^2  VectorParamsAs1DForOutWhenUnconnected=off
  wires:
  Product2/1 -> Reshape/1
  Centrifugal Moments/1((I * ω) x ω) -> Sum2/2
  Inertia Matrix/1 -> Product2/2
  Moments/1 -> Sum2/1
  Reshape1/1 -> Product2/1
  Demux1/1 -> Bus Creator1/1  "p"
  ωdot Integ/1 -> Demux1/1
  Demux1/3 -> Bus Creator1/3  "r"
  Demux1/2 -> Bus Creator1/2  "q"
  Bus Creator1/1 -> ω/1, Centrifugal Moments/1(ω)
  Sum2/1 -> Reshape1/1
  Reshape/1 -> Demux2/1, ωdot Integ/1
  Demux2/2 -> Bus Creator2/2  "qdot"
  Demux2/3 -> Bus Creator2/3  "rdot"
  Demux2/1 -> Bus Creator2/1  "pdot"
  Bus Creator2/1 -> ωdot/1

== system model_my_paper/Quadrotor/6DOF NWU Mixed/Quaternion Dynamics ==
  ω : Inport
  Another Rotational Dynamics : Subsystem
  Integrating : Subsystem
  Quat to Euler : Subsystem
  Quaternions to Direction Cosine Matrix : sharedtransform/Quaternions to  Direction Cosine Matrix  aMode=aMode
  qvec_dot : Subsystem
  DCM_be : Outport  OutDataTypeStr=double  VectorParamsAs1DForOutWhenUnconnected=off
  Quat : Outport  Port=2  OutDataTypeStr=double  VectorParamsAs1DForOutWhenUnconnected=off
  Euler : Outport  Port=3  OutDataTypeStr=double  VectorParamsAs1DForOutWhenUnconnected=off
  Rbe : Outport  Port=4  OutDataTypeStr=double  VectorParamsAs1DForOutWhenUnconnected=off
  wires:
  Integrating/1(Quat) -> Quaternions to Direction Cosine Matrix/1, Quat to Euler/1(q), qvec_dot/2(q), Quat/1
  Quaternions to Direction Cosine Matrix/1 -> DCM_be/1
  qvec_dot/1(qdot) -> Integrating/1(qdot)
  Quat to Euler/1(euler) -> Euler/1
  ω/1 -> Another Rotational Dynamics/1(w), qvec_dot/1(ω)
  Another Rotational Dynamics/1(Rbe) -> Rbe/1

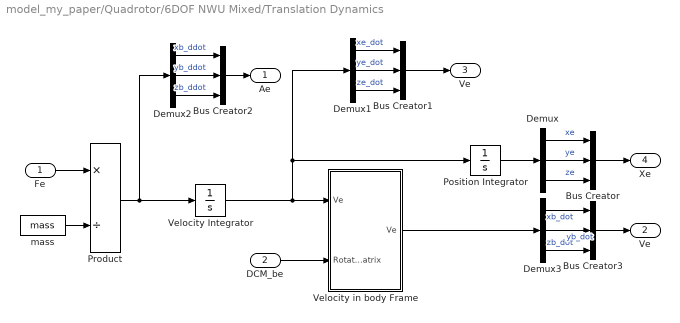
== system model_my_paper/Quadrotor/6DOF NWU Mixed/Translation Dynamics ==
  Fe : Inport
  DCM_be : Inport  Port=2
  Bus Creator{,1..3} (4 alike) : BusCreator  Inputs=3
  Demux{,1..3} (4 alike) : Demux  Outputs=3
  Position Integrator : Integrator  InitialCondition=PositionReferenceInitialValues  ContinuousStateAttributes={'xr', 'ye', 'ze'}
  Product : Product  Inputs=*/
  Velocity Integrator : Integrator  InitialCondition=VelocityBodyInitialValues  ContinuousStateAttributes={'u', 'v', 'w'}
  Velocity in body Frame : Subsystem
  mass : Constant  Value=mass
  Ae : Outport  OutDataTypeStr=double  Unit=m/s^2  VectorParamsAs1DForOutWhenUnconnected=off
  "Ve " : Outport  Port=2  OutDataTypeStr=double  Unit=m/s  VectorParamsAs1DForOutWhenUnconnected=off
  Ve : Outport  Port=3  OutDataTypeStr=double  Unit=m/s  VectorParamsAs1DForOutWhenUnconnected=off
  Xe : Outport  Port=4
  wires:
  mass/1 -> Product/2
  Demux/2 -> Bus Creator/2  "ye"
  Demux1/2 -> Bus Creator1/2  "ye_dot"
  Bus Creator/1 -> Xe/1
  Demux/1 -> Bus Creator/1  "xe"
  Position Integrator/1 -> Demux/1
  Demux/3 -> Bus Creator/3  "ze"
  Demux1/3 -> Bus Creator1/3  "ze_dot"
  Demux1/1 -> Bus Creator1/1  "xe_dot"
  DCM_be/1 -> Velocity in body Frame/2(Rotation Matrix)
  Velocity Integrator/1 -> Position Integrator/1, Demux1/1, Velocity in body Frame/1("Ve ")
  Demux2/3 -> Bus Creator2/3  "zb_ddot"
  Bus Creator2/1 -> Ae/1
  Demux2/2 -> Bus Creator2/2  "yb_ddot"
  Demux2/1 -> Bus Creator2/1  "xb_ddot"
  Bus Creator1/1 -> Ve/1
  Demux3/1 -> Bus Creator3/1  "xb_dot"
  Demux3/3 -> Bus Creator3/3  "zb_dot"
  Demux3/2 -> Bus Creator3/2  "yb_dot"
  Bus Creator3/1 -> "Ve "/1
  Product/1 -> Velocity Integrator/1, Demux2/1
  Fe/1 -> Product/1
  Velocity in body Frame/1(Ve) -> Demux3/1

== system model_my_paper/Quadrotor/Forces in Inertia frame/Gravity Force in Inertia Frame ==
  Mux1 : Mux  Inputs=3
  Reshape : Reshape  OutputDimensionality=Column vector (2-D)
  Unary Minus1 : UnaryMinus
  g : Gain  Gain=Gravity
  m : Constant  Value=mass
  x : Constant  Value=0
  y : Constant  Value=0
  Ge : Outport
  wires:
  Reshape/1 -> Ge/1
  g/1 -> Unary Minus1/1
  m/1 -> g/1
  y/1 -> Mux1/2
  Mux1/1 -> Reshape/1
  x/1 -> Mux1/1
  Unary Minus1/1 -> Mux1/3

== system model_my_paper/Quadrotor/Forces in Inertia frame/Thrust in Inertia Frame ==
  DCM_be : Inport
  Thrust : Inport  Port=2
  Mux1 : Mux  Inputs=3
  Product1 : Product  Multiplication=Matrix(*)  InputSameDT=on  SaturateOnIntegerOverflow=on  OutDataTypeStr=Inherit: Same as first input
  Reshape : Reshape  OutputDimensionality=Column vector (2-D)
  Transpose : Math  Operator=transpose
  x : Constant  Value=0
  y : Constant  Value=0
  Te : Outport
  wires:
  Mux1/1 -> Reshape/1
  y/1 -> Mux1/2
  DCM_be/1 -> Transpose/1
  Reshape/1 -> Product1/2
  Product1/1 -> Te/1
  x/1 -> Mux1/1
  Transpose/1 -> Product1/1
  Thrust/1 -> Mux1/3

== system model_my_paper/Rotation Dynamics Controller/Quaternion Dynamics/Euler Command ==
  q : Inport
  Bus Creator3 : BusCreator  Inputs=3
  Demux3 : Demux  Outputs=3
  Quaternions to Rotation Angles1 : sharedtransform/Quaternions to Rotation Angles  rotationOrder=ZYX  aMode=aMode
  Selector1 : Selector  InputPortWidth=3  IndexOptions=Index vector (dialog)  Indices=[3 2 1]  OutputSizes=1
  Unwrap : dspsigops/Unwrap  tol=pi  InputProcessing=Columns as channels (frame based)  running=off
  tag scope: Euler_c=global
  wires:
  q/1 -> Quaternions to Rotation Angles1/1
  Demux3/1 -> Bus Creator3/1  "ϕc"
  Quaternions to Rotation Angles1/1 -> Selector1/1
  Unwrap/1 -> Bus Creator3/3  "Ψd"
  Bus Creator3/1 -> [Euler_c]
  Demux3/3 -> Unwrap/1
  Selector1/1 -> Demux3/1
  Demux3/2 -> Bus Creator3/2  "θc"

== system model_my_paper/Rotation Dynamics Controller/Quaternion Dynamics/Euler Desired ==
  DCM : Inport
  Bus Creator1 : BusCreator  Inputs=3
  Demux1 : Demux  Outputs=3
  Direction Cosine Matrix to Rotation Angles : sharedtransform/Direction Cosine Matrix to Rotation Angles  rotationOrder=ZYX  aMode=aMode  action=None  tolerance=eps(2)
      settings: LibrarySourceBlock=|
      | aerolibtransform2/Direction Cosine Matrix
      | to Rotation Angles
  Selector : Selector  InputPortWidth=3  IndexOptions=Index vector (dialog)  Indices=[3 2 1]  OutputSizes=1
  Unwrap1 : dspsigops/Unwrap  tol=pi  InputProcessing=Columns as channels (frame based)  running=off
  tag scope: Euler_d=global
  wires:
  DCM/1 -> Direction Cosine Matrix to Rotation Angles/1
  Demux1/3 -> Unwrap1/1
  Demux1/1 -> Bus Creator1/1  "ϕd"
  Selector/1 -> Demux1/1
  Bus Creator1/1 -> [Euler_d]
  Unwrap1/1 -> Bus Creator1/3  "Ψd"
  Direction Cosine Matrix to Rotation Angles/1 -> Selector/1
  Demux1/2 -> Bus Creator1/2  "θd"

== system model_my_paper/Quadrotor/6DOF NWU Mixed/Angular Velocity Dyanmics/Centrifugal Moments ==
  ω : Inport
  3x3 Cross Product : sharedutil/3x3 Cross Product  aMode=aMode
  Inertia Matrix : Constant  Value=InertiaMatrix
  Product : Product  Multiplication=Matrix(*)  InputSameDT=on  SaturateOnIntegerOverflow=on  OutDataTypeStr=Inherit: Same as first input
  To1D : Reshape
  ToVec : Reshape  OutputDimensionality=Column vector (2-D)
  (I * ω) x ω : Outport
  wires:
  ToVec/1 -> Product/2
  Product/1 -> To1D/1
  Inertia Matrix/1 -> Product/1
  ω/1 -> 3x3 Cross Product/2, ToVec/1
  3x3 Cross Product/1 -> (I * ω) x ω/1
  To1D/1 -> 3x3 Cross Product/1  "I * ω"

== system model_my_paper/Quadrotor/6DOF NWU Mixed/Quaternion Dynamics/Another Rotational Dynamics ==
  w : Inport
  Integrator : Integrator  InitialCondition=eye(3)
  Matrix Multiply1 : Product  Multiplication=Matrix(*)
  Skew : Subsystem
  Unary Minus : UnaryMinus
  Rbe : Outport
  wires:
  Skew/1(Wx) -> Unary Minus/1
  Integrator/1 -> Rbe/1, Matrix Multiply1/2
  Unary Minus/1 -> Matrix Multiply1/1
  Matrix Multiply1/1 -> Integrator/1
  w/1 -> Skew/1(w)

== system model_my_paper/Quadrotor/6DOF NWU Mixed/Quaternion Dynamics/Integrating ==
  qdot : Inport
  Bus Creator1 : BusCreator  Inputs=q0,vec  OutDataTypeStr=Bus: QuaturnionBus
  Demux2 : Demux
  Initial Euler Angles : Constant  Value=EulerInitialValues
  Mux : Mux  Inputs=3
  Quaternion Integration : Integrator  InitialConditionSource=external  InitialCondition=[e0_0 e1_0 e2_0 e3_0]  ContinuousStateAttributes={'q0', 'q1', 'q2', 'q3'}
  Rotation Angles to Quaternions : sharedtransform/Rotation Angles to Quaternions  rotationOrder=ZYX  aMode=aMode
  Selector : Selector  InputPortWidth=3  IndexOptions=Index vector (dialog)  Indices=[3 2 1]  OutputSizes=1
  Quat : Outport  OutDataTypeStr=double  VectorParamsAs1DForOutWhenUnconnected=off
  wires:
  Initial Euler Angles/1 -> Selector/1
  Rotation Angles to Quaternions/1 -> Quaternion Integration/2
  Selector/1 -> Rotation Angles to Quaternions/1
  qdot/1 -> Quaternion Integration/1
  Quaternion Integration/1 -> Demux2/1
  Demux2/2 -> Mux/1
  Demux2/4 -> Mux/3
  Bus Creator1/1 -> Quat/1
  Demux2/3 -> Mux/2
  Mux/1 -> Bus Creator1/2  "vec"
  Demux2/1 -> Bus Creator1/1  "q0"

== system model_my_paper/Quadrotor/6DOF NWU Mixed/Quaternion Dynamics/Quat to Euler ==
  q : Inport
  Bus Creator3 : BusCreator  Inputs=3
  Demux3 : Demux  Outputs=3
  Quaternions to Rotation Angles : sharedtransform/Quaternions to Rotation Angles  rotationOrder=ZYX  aMode=aMode
  Selector : Selector  InputPortWidth=3  IndexOptions=Index vector (dialog)  Indices=[3 2 1]  OutputSizes=1
  Unwrap2 : dspsigops/Unwrap  tol=pi  InputProcessing=Columns as channels (frame based)  running=off
  euler : Outport
  wires:
  Quaternions to Rotation Angles/1 -> Selector/1
  q/1 -> Quaternions to Rotation Angles/1
  Selector/1 -> Demux3/1
  Bus Creator3/1 -> euler/1
  Demux3/2 -> Bus Creator3/2  "θ"
  Demux3/1 -> Bus Creator3/1  "ϕ"
  Demux3/3 -> Unwrap2/1  "Ψ"
  Unwrap2/1 -> Bus Creator3/3  "Ψ"

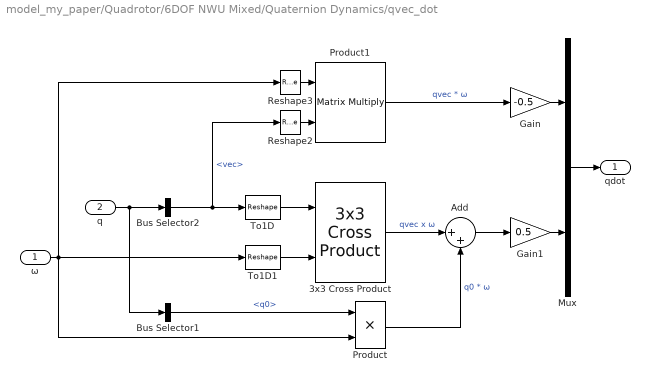
== system model_my_paper/Quadrotor/6DOF NWU Mixed/Quaternion Dynamics/qvec_dot ==
  ω : Inport  OutDataTypeStr=double
  q : Inport  Port=2
  3x3 Cross Product : sharedutil/3x3 Cross Product  aMode=aMode
  Add : Sum  Inputs=|++
  Bus Selector1 : BusSelector  OutputSignals=q0
  Bus Selector2 : BusSelector  OutputSignals=vec
  Gain : Gain  Gain=-0.5
  Gain1 : Gain  Gain=0.5
  Mux : Mux  Inputs=2
  Product : Product
  Product1 : Product  Inputs=**  Multiplication=Matrix(*)  SaturateOnIntegerOverflow=on  OutDataTypeStr=Inherit: Same as first input
  Reshape2 : Reshape  OutputDimensionality=Column vector (2-D)
  Reshape3 : Reshape  OutputDimensionality=Row vector (2-D)
  To1D : Reshape
  To1D1 : Reshape
  qdot : Outport
  wires:
  Add/1 -> Gain1/1
  Bus Selector1/1 -> Product/1  "<q0>"
  To1D1/1 -> 3x3 Cross Product/2
  To1D/1 -> 3x3 Cross Product/1
  Bus Selector2/1 -> Reshape2/1, To1D/1  "<vec>"
  3x3 Cross Product/1 -> Add/1  "qvec x ω"
  Product/1 -> Add/2  "q0 * ω"
  Gain1/1 -> Mux/2
  q/1 -> Bus Selector1/1, Bus Selector2/1
  Reshape3/1 -> Product1/1
  Product1/1 -> Gain/1  "qvec * ω"
  ω/1 -> To1D1/1, Product/2, Reshape3/1
  Gain/1 -> Mux/1
  Reshape2/1 -> Product1/2
  Mux/1 -> qdot/1

== system model_my_paper/Quadrotor/6DOF NWU Mixed/Translation Dynamics/Velocity in body Frame ==
  "Ve " : Inport
  Rotation Matrix : Inport  Port=2
  Product1 : Product  Multiplication=Matrix(*)  InputSameDT=on  SaturateOnIntegerOverflow=on  OutDataTypeStr=Inherit: Same as first input
  Reshape1 : Reshape  OutputDimensionality=Column vector (2-D)
  Reshape2 : Reshape
  Ve : Outport  VectorParamsAs1DForOutWhenUnconnected=off
  wires:
  "Ve "/1 -> Reshape1/1
  Reshape1/1 -> Product1/2
  Product1/1 -> Reshape2/1
  Reshape2/1 -> Ve/1
  Rotation Matrix/1 -> Product1/1

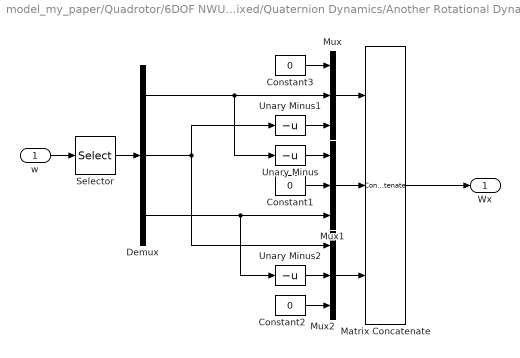
== system model_my_paper/Quadrotor/6DOF NWU Mixed/Quaternion Dynamics/Another Rotational Dynamics/Skew ==
  w : Inport
  Constant1 : Constant  Value=0
  Constant2 : Constant  Value=0
  Constant3 : Constant  Value=0
  Demux : Demux  Outputs=3
  Matrix Concatenate : Concatenate  NumInputs=3  Mode=Multidimensional array  ConcatenateDimension=2
  Mux : Mux  Inputs=3
  Mux1 : Mux  Inputs=3
  Mux2 : Mux  Inputs=3
  Selector : Selector  InputPortWidth=3  IndexOptions=Index vector (dialog)  Indices=[3 2 1]  OutputSizes=1
  Unary Minus : UnaryMinus
  Unary Minus1 : UnaryMinus
  Unary Minus2 : UnaryMinus
  Wx : Outport
  wires:
  Constant2/1 -> Mux2/3
  Demux/1 -> Unary Minus/1, Mux/2
  Unary Minus/1 -> Mux1/1
  Constant3/1 -> Mux/1
  Demux/3 -> Unary Minus2/1, Mux1/3
  Demux/2 -> Unary Minus1/1, Mux2/1
  Unary Minus2/1 -> Mux2/2
  Constant1/1 -> Mux1/2
  Mux1/1 -> Matrix Concatenate/2
  Mux/1 -> Matrix Concatenate/1
  Mux2/1 -> Matrix Concatenate/3
  Unary Minus1/1 -> Mux/3
  Matrix Concatenate/1 -> Wx/1
  Selector/1 -> Demux/1
  w/1 -> Selector/1

== matlab function model_my_paper/Rotation Dynamics Controller/My paper controller/MATLAB Function ==
  data: sr output size=[3 1]; sw output size=[3 1]; wc output size=[3 1]; qw output size=[3 1]; Kr input size=[3 3]; Kw input size=[3 3]; wd_dot output size=[3 1]; R input size=[3 3]; w input size=[3 1]; Rd input size=[3 3]; Rd_dot input size=[3 3]; wd input size=[3 1]
function [sr, sw, wc, qw, wd_dot] = fcn(Kr, Kw, R, w, Rd, Rd_dot, wd)

% sR = Rd' * R - eye(3);
% sr = InvSkew(sR);
% wc = Kr * sr;

Re = Rd * R';
sr = 0.5 * InvSkew(Re - Re');

RdR = Rd_dot' * R;
W1 = 0.5 * InvSkew(RdR - RdR');
W2 = 0.5 * (eye(3) * trace(Re') - Re');
wc = W2 \ (-W1 - Kr * sr);

Tau_w = 35;
wd_dot = Tau_w * (wc-wd);

%sw = w - Re * wd;
% alpha = -Skew(w) * Re' * wd + Re' * wd_dot;

sw = w - wd;
alpha = wd_dot;
qw = alpha - Kw * sw;

function mat = Skew(vec)
    mat = [0, -vec(3), vec(2); vec(3), 0, -vec(1); -vec(2), vec(1), 0];
end

function vec = InvSkew(mat)
    vec = zeros(3, 1);
    vec(1) = (mat(3,2) - mat(2,3)) / 2;
    vec(2) = (mat(1,3) - mat(3,1)) / 2;
    vec(3) = (mat(2,1) - mat(1,2)) / 2;
end
end

== matlab function model_my_paper/Translation Dynamics Controller/My paper Translation Controller but for Quaternion/MATLAB Function ==
  data: ep output size=[3 1]; ev output size=[3 1]; s output size=[3 1]; U output size=[3 1]; Fth output size=1; qc_0 output size=1; Kx input size=[3 3]; Kv input size=[3 3]; x input size=[3 1]; v input size=[3 1]; xd input size=[3 1]; vd input size=[3 1]; ad input size=[3 1]; mass input size=1; qc_vec output size=[1 3]
function [ep, ev, s, U, Fth, qc_0, qc_vec] = fcn(Kx, Kv, x, v, xd, vd, ad, mass)

g = 9.81;

ep = x - xd;
ev = v - vd;
s = ev + Kx * ep;
U = ad - Kx * ev - Kv * s;

Fth = mass * sqrt(U(1)^2 + U(2)^2 + (U(3) + g)^2);

q0 = sqrt((mass * (g + U(3)) / (2 * Fth)) + 1/2);
vec = [-mass * U(2) / 2 / Fth / q0,...
        mass * U(1) / 2 / Fth / q0,...
                                  0];
n = sqrt(q0^2 + vec(1)^2 + vec(2)^2 + vec(3)^2);
qc_0 = q0/n;
qc_vec = vec/n;

Fth = mass * (U(3) + g);

end
